simulink model "HILModel"  (Simulink 6.6)
settings: Solver=ode4  StartTime=0.0  StopTime=20  FixedStep=SampleT  RelTol=1e-3
InitFcn:
  | clc
  | Taxi_Var_new
  | failures
  | insInit
  | piccolo_init
values from neighbouring files (symbols this model uses):
  A1 = 0    [Taxi_Var.m]
  Apolar = 0.0899    [Taxi_Var.m]
  CD0 = 0.0219    [Taxi_Var.m]
  chord = S/span    (= 0.384036716878)    [Taxi_Var.m]
  CL0 = 0.1857    [Taxi_Var.m]
  CLa = 4.6206    [Taxi_Var.m]
  CLa_dot = 1.93    [Taxi_Var.m]
  Clb = -0.0043    [Taxi_Var.m]
  ClDa = 0.1695    [Taxi_Var.m]
  CLDe = 0.4032    [Taxi_Var.m]
  CLDf = 0.047    [Taxi_Var.m]
  ClDr = 0.0003    [Taxi_Var.m]
  Clp = -0.4425    [Taxi_Var.m]
  CLq = 8.7465    [Taxi_Var.m]
  Clr = 0.0675    [Taxi_Var.m]
  Cm0 = -0.0902    [Taxi_Var.m]
  Cma = -1.3995    [Taxi_Var.m]
  CmDe = -0.9493    [Taxi_Var.m]
  CmDf = -.021    (= -0.021)    [Taxi_Var.m]
  Cmq = -10.8760    (= -10.876)    [Taxi_Var.m]
  Cnb = 0.0281    [Taxi_Var.m]
  CnDa = -0.0031    [Taxi_Var.m]
  CnDr = -0.0882    [Taxi_Var.m]
  Cnp = -0.0695    [Taxi_Var.m]
  Cnr = -0.1045    [Taxi_Var.m]
  CYb = -0.1999    [Taxi_Var.m]
  CYDr = 0.0192    [Taxi_Var.m]
  damax = 25*deg2rad    (= 0.436332312999)    [Taxi_Var.m]
  damin = -25*deg2rad    (= -0.436332312999)    [Taxi_Var.m]
  datrim = 0*deg2rad    (= 0)    [Taxi_Var.m]
  demax = 15*deg2rad    (= 0.261799387799)    [Taxi_Var.m]
  demin = -15*deg2rad    (= -0.261799387799)    [Taxi_Var.m]
  detrim = -2.4137*deg2rad    (= -0.0421270121554)    [Taxi_Var.m]
  dfland = 30*deg2rad    (= 0.523598775598)    [Taxi_Var.m]
  dfmax = 30*deg2rad    (= 0.523598775598)    [Taxi_Var.m]
  dfmin = 0*deg2rad    (= 0)    [Taxi_Var.m]
  drmax = 25*deg2rad    (= 0.436332312999)    [Taxi_Var.m]
  drmin = -25*deg2rad    (= -0.436332312999)    [Taxi_Var.m]
  drtrim = 0*deg2rad    (= 0)    [Taxi_Var.m]
  dtmax = 1    [Taxi_Var.m]
  dtmin = 0    [Taxi_Var.m]
  dttrim = 0.0725    [Taxi_Var.m]
  Euler_0 = [0; 0; 45]'*pi/180    [Taxi_Var.m]    (also in hilInit.m = [0; 0; 0*pi/180]')
  ISA_g = 9.815    [Taxi_Var.m]
  ISA_hmax = 2000    [Taxi_Var.m]
  ISA_lapse = .0065    (= 0.0065)    [Taxi_Var.m]
  ISA_P0 = 101325    [Taxi_Var.m]
  ISA_R = 287    [Taxi_Var.m]
  ISA_rho0 = 1.225    [Taxi_Var.m]
  ISA_T0 = 289    [Taxi_Var.m]
  Ixx = 3.689084    [Taxi_Var.m]
  Iyy = 7.43789    [Taxi_Var.m]
  Izz = 10.22202    [Taxi_Var.m]
  mass = 22.5    [Taxi_Var.m]
  MinThK = 0.075    [Taxi_Var.m]
  Pos_0 = [0; 0; 1000]'    [Taxi_Var.m]    (also in hilInit.m = [500; 750; 350]')
  PQR_0 = [0; 0; 0]'    [Taxi_Var.m]
  span = 2.3368    [Taxi_Var.m]
  TFact = 0.4    [Taxi_Var.m]
  ThK = 2.18    [Taxi_Var.m]
  Vb_0 = [35; 0; 0]'    [Taxi_Var.m]
undefined symbols (not defined in the file or in its folder): clock, Earth, IdxCmdOrbitRadius, IdxCmdOrbitSense, IdxCmdWp1Alt, IdxCmdWp1Lat, IdxCmdWp1Lon, IdxCmdWp2Alt, IdxCmdWp2Lat, IdxCmdWp2Lon, IdxEstimReserved1, IdxEstimWEast, IdxEstimWNorth, IdxGainsAltD, IdxGainsAltI, IdxGainsAltP, IdxGainsPdynD, IdxGainsPdynI, IdxGainsPdynP, IdxGainsPitchD, IdxGainsPitchI, IdxGainsPitchP, IdxGainsRollD, IdxGainsRollI, IdxGainsRollP, IdxGainsSlopeElevatorD, IdxGainsSlopeElevatorP, IdxGainsTrackConv, IdxGainsTrackD, IdxGainsTrackI, IdxGainsTrackP, IdxGainsTurnD, IdxGainsTurnI, IdxGainsTurnP, IdxGainsYawD, IdxGainsYawI, IdxGainsYawP, IdxLimitsAileronMax, IdxLimitsAileronMin, IdxLimitsBankMax, IdxLimitsBankMin, IdxLimitsElevatorMax, IdxLimitsElevatorMin, IdxLimitsFlapMax, IdxLimitsFlapMin, IdxLimitsPdynMax, IdxLimitsPdynMin, IdxLimitsRudderMax, IdxLimitsRudderMin, IdxLimitsThrottleMax, IdxLimitsThrottleMin, IdxSensorsAlt, IdxSensorsLat, IdxSensorsLon, IdxSensorsVDown, IdxSensorsVEast, IdxSensorsVNorth, IdxStatesGlobal, IdxStatesManual, IdxStatesMode ... (+3)
libraries: piccolo_library x60, simulink x32, aerolibasang x5, aerolibconvert2 x5, aerosimlib x3, aerolibtransform2 x2, aerolibnav x2, xpclib x1, aerolibatmos2 x1, dspmtrx3 x1
(part 3 of 4)

== system HILModel/Autopilot/Autopilot/Altitude Control Vector Inputs/Integral Gain  Scheduling ==
  note: 3. Then the IntegralGain2 = IntegralGain * GainScheduleFactor
  note: 2. We compute GainScheduleFactor = exp(-error^2 / (2*sigma^2))
  note: 1. We compute sigma = ScalingParam * ActuatorRange/2 / Kp
  note: Integral gain scheduling based on a Gaussian distribution, as a function of the error, actuator range, and proportional gain.
  err : Inport
  Gains : Inport  Port=2
  Limits : Inport  Port=3
  Demux : Demux  Outputs=2
  Demux1 : Demux  Outputs=3
  Gain : Gain  Gain=0.5  SaturateOnIntegerOverflow=on
  Gain1 : Gain  Gain=2  SaturateOnIntegerOverflow=on
  Gain2 : Gain  Gain=-1  SaturateOnIntegerOverflow=on
  Math Function : Math  Operator=square  OutDataType=fixdt(1,16,0)  OutScaling=[]  SaturateOnIntegerOverflow=on
  Math Function1 : Math  Operator=square  OutDataType=fixdt(1,16,0)  OutScaling=[]  SaturateOnIntegerOverflow=on
  Math Function2 : Math  OutDataType=fixdt(1,16,0)  OutScaling=[]  SaturateOnIntegerOverflow=on
  Mux1 : Mux  Inputs=3
  Product : Product  Inputs=/**  SaturateOnIntegerOverflow=on
  Product1 : Product  Inputs=*/  SaturateOnIntegerOverflow=on
  Product2 : Product  SaturateOnIntegerOverflow=on
  Scaling param : Constant  Value=0.5
  Sum : Sum  Inputs=+-  SaturateOnIntegerOverflow=on
  Zero Protect : piccolo_library/Math/Zero Protect  SystemSampleTime=-1  p=1  tol=1e-6
  Gains2 : Outport  OutDataType=fixdt(1,16,0)  OutScaling=[]
  wires:
  Zero Protect/1 -> Product/1
  Demux1/1 -> Mux1/1, Zero Protect/1
  Demux1/3 -> Mux1/3
  Product2/1 -> Mux1/2
  Mux1/1 -> Gains2/1
  Demux1/2 -> Product2/2
  Gains/1 -> Demux1/1
  Math Function2/1 -> Product2/1
  Product1/1 -> Math Function2/1
  Gain1/1 -> Product1/2
  Gain2/1 -> Product1/1
  Math Function1/1 -> Gain2/1
  err/1 -> Math Function1/1
  Math Function/1 -> Gain1/1
  Product/1 -> Math Function/1
  Scaling param/1 -> Product/3
  Gain/1 -> Product/2
  Sum/1 -> Gain/1
  Demux/2 -> Sum/2
  Demux/1 -> Sum/1
  Limits/1 -> Demux/1

== system HILModel/Autopilot/Autopilot/Altitude Control Vector Inputs/Min alt ==
  note: Determin the min altitude to use. Either -10000 or the passed in value, depending on if Auto land is enabled
  Globals : Inport
  MinAlt : Inport  Port=2
  -10000 : Constant  Value=-10000
  Climbout : Constant  Value=0
  Convert to 1 based : Constant  Value=1.1
  Default : Constant  Value=0
  Demux : Demux  Outputs=3
  Final Approach : Constant
  Flying : Constant  Value=0
  Land pattern : Constant
  Loop on or off : Switch  Threshold=0.5  SaturateOnIntegerOverflow=on
  Min alt on/off : MultiPortSwitch  Inputs=8  SaturateOnIntegerOverflow=on  InputSameDT=on
  Pre launch : Constant  Value=0
  Sum : Sum  Inputs=++|  SaturateOnIntegerOverflow=on  InputSameDT=on
  Terminator : Terminator
  Terminator1 : Terminator
  Touchdown : Constant
  Transition : Constant  Value=0
  MinAltOut : Outport  OutDataType=fixdt(1,16,0)  OutScaling=[]
  wires:
  Sum/1 -> Min alt on/off/1
  Default/1 -> Min alt on/off/9
  Touchdown/1 -> Min alt on/off/8
  Final Approach/1 -> Min alt on/off/7
  Land pattern/1 -> Min alt on/off/6
  Flying/1 -> Min alt on/off/5
  Transition/1 -> Min alt on/off/3
  Climbout/1 -> Min alt on/off/4
  Pre launch/1 -> Min alt on/off/2
  -10000/1 -> Loop on or off/1
  Min alt on/off/1 -> Loop on or off/2
  Loop on or off/1 -> MinAltOut/1
  Globals/1 -> Demux/1
  Demux/1 -> Terminator1/1
  MinAlt/1 -> Loop on or off/3
  Demux/2 -> Sum/2
  Convert to 1 based/1 -> Sum/1
  Demux/3 -> Terminator/1

== system HILModel/Autopilot/Autopilot/Altitude Control Vector Inputs/PID Controller ==
  note: Standard PID feedback controller with integrator saturation. There are three gains, and three states, one for each term
  Input : Inport
  Cmd : Inport  Port=2
  State : Inport  Port=3
  Gains : Inport  Port=4
  Limits : Inport  Port=5
  IniCond : Inport  Port=6
  Demux : Demux  Outputs=3
  Demux1 : Demux  Outputs=3
  Derivative Gain : Product  Inputs=3  SaturateOnIntegerOverflow=on  InputSameDT=on
  Extended Integrator : Subsystem  AncestorBlock=piccolo_library/Integrators/Extended Integrator  mask(Extended Integrator){T=tsamp}
      mask prompts: T "Sample time:"
      mask help:
      | Trapezoidal integration with integrator reset and anti-windup logic
      | The block computes the integral.  The integrator gets the IC value
      | whenever the enable line is down.  Anytime the enable line is
      | down the output is the IC value.  If the gain goes to zero then the
      | integrator value is reset.
  Proportional Gain : Product  Inputs=3  SaturateOnIntegerOverflow=on  InputSameDT=on
  Scope1 : Scope  NumInputPorts=3
      settings: YMin=0.045~0.038~-1  YMax=0.051~0.058~1  SaveName=ScopeData32
  Scope2 : Scope  NumInputPorts=3
      settings: YMin=0.045~0.038~-1  YMax=0.051~0.058~1  SaveName=ScopeData20
  Sum : Sum  Inputs=|+-  SaturateOnIntegerOverflow=on
  Sum3 : Sum  Inputs=+++  SaturateOnIntegerOverflow=on  InputSameDT=on
  dx/dt with TD : piccolo_library/Derivatives/dx//dt with TD  SystemSampleTime=-1  tsamp=tsamp  tdelay=tdelay
  Output : Outport  OutDataType=fixdt(1,16,0)  OutScaling=[]
  wires:
  Sum3/1 -> Output/1
  Demux1/3 -> Derivative Gain/3
  Demux1/2 -> Extended Integrator/3(Enable)
  Demux1/1 -> Proportional Gain/3
  State/1 -> Demux1/1
  IniCond/1 -> Extended Integrator/2(IniCond)
  Limits/1 -> Extended Integrator/5(Limits)
  Demux/2 -> Extended Integrator/4(Gain)
  Extended Integrator/1(Out) -> Sum3/2, Scope2/2
  Derivative Gain/1 -> Sum3/3, Scope2/3
  Proportional Gain/1 -> Sum3/1, Scope2/1
  Demux/3 -> Derivative Gain/2
  Demux/1 -> Proportional Gain/2
  Gains/1 -> Demux/1
  dx/dt with TD/1 -> Derivative Gain/1
  Sum/1 -> Extended Integrator/1(Input), dx/dt with TD/1, Proportional Gain/1
  Cmd/1 -> Sum/2, Scope1/1, Scope1/2
  Input/1 -> Sum/1

== system HILModel/Autopilot/Autopilot/Altitude Control Vector Inputs/Total Energy1 ==
  TAS : Inport
  Alt : Inport  Port=2
  TASCmd : Inport  Port=3
  AltCmd : Inport  Port=4
  State : Inport  Port=5
  1/2 : Constant  Value=0.5
  Kinetic : Product  Inputs=***  SaturateOnIntegerOverflow=on  InputSameDT=on
  Kinetic1 : Product  Inputs=*/  SaturateOnIntegerOverflow=on  InputSameDT=on
  Kinetic2 : Product  Inputs=***  SaturateOnIntegerOverflow=on  InputSameDT=on
  Sum1 : Sum  SaturateOnIntegerOverflow=on  InputSameDT=on
  Sum2 : Sum  SaturateOnIntegerOverflow=on  InputSameDT=on
  Switch : Switch  Threshold=0.5  SaturateOnIntegerOverflow=on
  Switch1 : Switch  Threshold=0.5  SaturateOnIntegerOverflow=on
  Zero : Constant  Value=0.0
  g1 : Constant  Value=9.806
  Energy : Outport  OutDataType=fixdt(1,16,0)  OutScaling=[]
  Cmd : Outport  Port=2  OutDataType=fixdt(1,16,0)  OutScaling=[]
  wires:
  TASCmd/1 -> Kinetic2/3, Kinetic2/2
  Sum1/1 -> Cmd/1
  AltCmd/1 -> Sum1/2
  Switch1/1 -> Sum1/1
  Kinetic2/1 -> Switch1/1
  Sum2/1 -> Energy/1
  Alt/1 -> Sum2/1
  Switch/1 -> Sum2/2
  Kinetic1/1 -> Kinetic2/1, Kinetic/3
  1/2/1 -> Kinetic1/1
  g1/1 -> Kinetic1/2
  Kinetic/1 -> Switch/1
  State/1 -> Switch/2, Switch1/2
  Zero/1 -> Switch/3, Switch1/3
  TAS/1 -> Kinetic/1, Kinetic/2

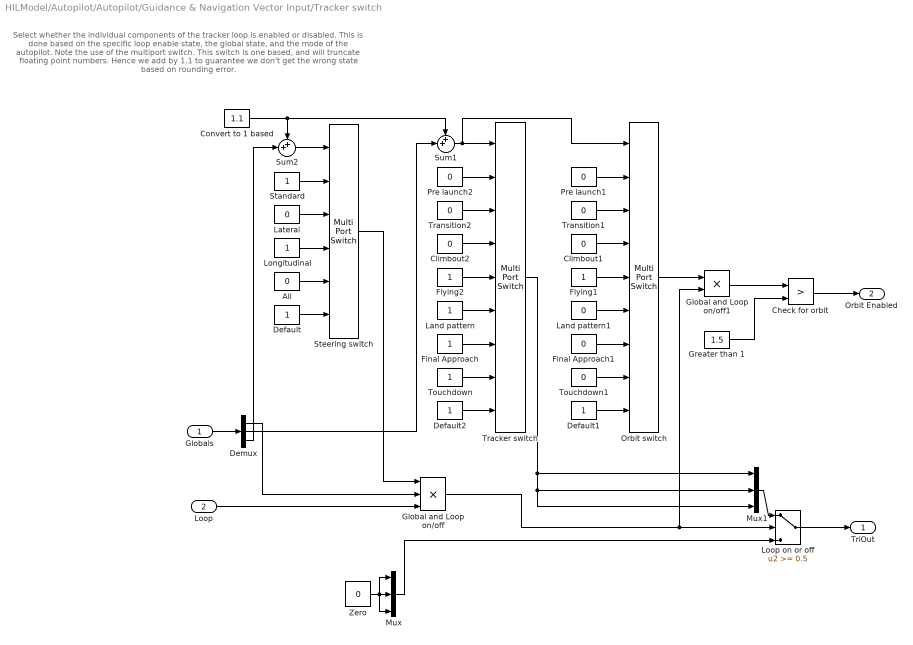
== system HILModel/Autopilot/Autopilot/Guidance & Navigation Vector Input/Tracker switch ==
  note: Select whether the individual components of the tracker loop is enabled or
      | disabled.  This is done based on the specific loop enable state, the global state, and the mode of the autopilot.
      |
      | Note the use of the multiport  switch.  This switch is one based, and will truncate floating point
      | numbers.  Hence we add by 1.1 to guarantee we don't get the wrong state based on rounding
      | error.
  Globals : Inport
  Loop : Inport  Port=2
  All : Constant  Value=0
  Check for orbit : RelationalOperator  Operator=>
  Climbout1 : Constant  Value=0
  Climbout2 : Constant  Value=0
  Convert to 1 based : Constant  Value=1.1
  Default : Constant
  Default1 : Constant
  Default2 : Constant
  Demux : Demux  Outputs=3
  Final Approach : Constant
  Final Approach1 : Constant  Value=0
  Flying1 : Constant
  Flying2 : Constant
  Global and Loop on/off : Product  Inputs=3  SaturateOnIntegerOverflow=on
  Global and Loop on/off1 : Product  SaturateOnIntegerOverflow=on
  Greater than 1 : Constant  Value=1.5
  Land pattern : Constant
  Land pattern1 : Constant  Value=0
  Lateral : Constant  Value=0
  Longitudinal : Constant
  Loop on or off : Switch  Threshold=0.5  SaturateOnIntegerOverflow=on
  Mux : Mux  Inputs=3
  Mux1 : Mux  Inputs=3
  Orbit switch : MultiPortSwitch  Inputs=8  SaturateOnIntegerOverflow=on  InputSameDT=on
  Pre launch1 : Constant  Value=0
  Pre launch2 : Constant  Value=0
  Standard : Constant
  Steering switch : MultiPortSwitch  Inputs=5  SaturateOnIntegerOverflow=on  InputSameDT=on
  Sum1 : Sum  Inputs=++|  SaturateOnIntegerOverflow=on  InputSameDT=on
  Sum2 : Sum  Inputs=++|  SaturateOnIntegerOverflow=on  InputSameDT=on
  Touchdown : Constant
  Touchdown1 : Constant  Value=0
  Tracker switch : MultiPortSwitch  Inputs=8  SaturateOnIntegerOverflow=on  InputSameDT=on
  Transition1 : Constant  Value=0
  Transition2 : Constant  Value=0
  Zero : Constant  Value=0
  TriOut : Outport  OutDataType=fixdt(1,16,0)  OutScaling=[]
  Orbit Enabled : Outport  Port=2  OutDataType=fixdt(1,16,0)  OutScaling=[]
  wires:
  Steering switch/1 -> Global and Loop on/off/1
  Demux/1 -> Global and Loop on/off/2
  Loop/1 -> Global and Loop on/off/3
  Sum2/1 -> Steering switch/1
  Default/1 -> Steering switch/6
  All/1 -> Steering switch/5
  Lateral/1 -> Steering switch/3
  Longitudinal/1 -> Steering switch/4
  Standard/1 -> Steering switch/2
  Convert to 1 based/1 -> Sum2/1, Sum1/1
  Default1/1 -> Orbit switch/9
  Touchdown1/1 -> Orbit switch/8
  Final Approach1/1 -> Orbit switch/7
  Land pattern1/1 -> Orbit switch/6
  Flying1/1 -> Orbit switch/5
  Transition1/1 -> Orbit switch/3
  Climbout1/1 -> Orbit switch/4
  Pre launch1/1 -> Orbit switch/2
  Sum1/1 -> Orbit switch/1, Tracker switch/1
  Default2/1 -> Tracker switch/9
  Touchdown/1 -> Tracker switch/8
  Final Approach/1 -> Tracker switch/7
  Land pattern/1 -> Tracker switch/6
  Flying2/1 -> Tracker switch/5
  Transition2/1 -> Tracker switch/3
  Climbout2/1 -> Tracker switch/4
  Pre launch2/1 -> Tracker switch/2
  Mux1/1 -> Loop on or off/1
  Tracker switch/1 -> Mux1/2, Mux1/3, Mux1/1
  Zero/1 -> Mux/3, Mux/2, Mux/1
  Mux/1 -> Loop on or off/3
  Check for orbit/1 -> Orbit Enabled/1
  Greater than 1/1 -> Check for orbit/2
  Orbit switch/1 -> Global and Loop on/off1/1
  Global and Loop on/off1/1 -> Check for orbit/1
  Demux/3 -> Sum2/2
  Demux/2 -> Sum1/2
  Global and Loop on/off/1 -> Global and Loop on/off1/2, Loop on or off/2
  Globals/1 -> Demux/1
  Loop on or off/1 -> TriOut/1

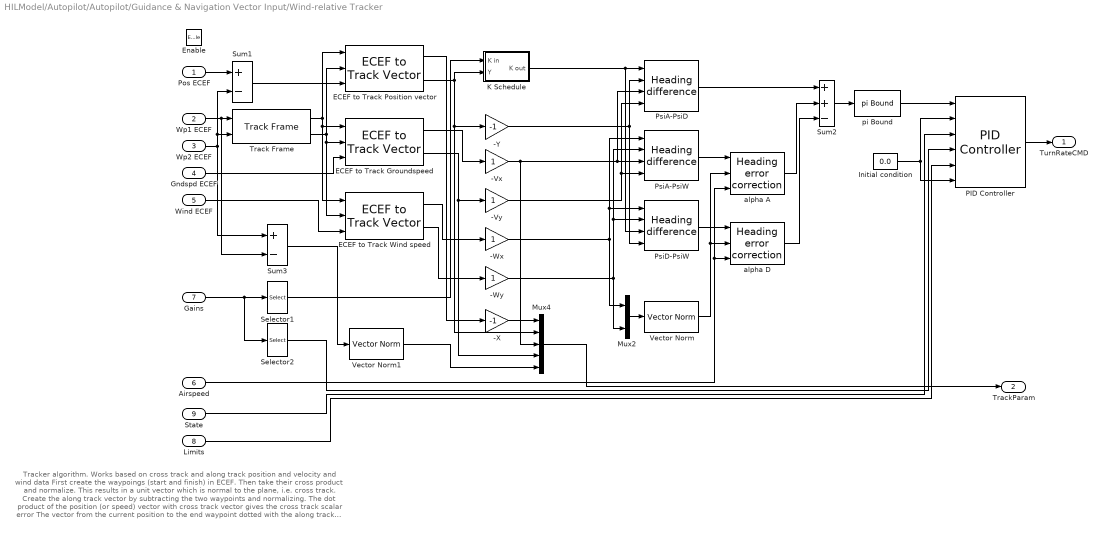
== system HILModel/Autopilot/Autopilot/Guidance & Navigation Vector Input/Wind-relative Tracker ==
  note: Tracker algorithm.  Works based on cross track and along track position and velocity and wind data
      |
      | First create the waypoings (start and finish) in ECEF.  Then take their cross product and normalize.  This results in a unit vector which is normal to the plane, i.e. cross track.
      | Create the along track vector by subtracting the two waypoints and normalizing.
      | The dot product of the position (or speed) vector with cross track vector gives the cross track scalar error
      | The vector from the current position to the end waypoint dotted with the along track vector gives the along track value
  Pos ECEF : Inport
  Wp1 ECEF : Inport  Port=2
  Wp2 ECEF : Inport  Port=3
  Gndspd ECEF : Inport  Port=4
  Wind ECEF : Inport  Port=5
  Airspeed : Inport  Port=6
  Gains : Inport  Port=7
  Limits : Inport  Port=8
  State : Inport  Port=9
  Enable : EnablePort
  -Vx : Gain  SaturateOnIntegerOverflow=on
  -Vy : Gain  SaturateOnIntegerOverflow=on
  -Wx : Gain  SaturateOnIntegerOverflow=on
  -Wy : Gain  SaturateOnIntegerOverflow=on
  -X : Gain  Gain=-1  SaturateOnIntegerOverflow=on
  -Y : Gain  Gain=-1  SaturateOnIntegerOverflow=on
  ECEF to Track Groundspeed : piccolo_library/Transformations/ECEF to Track Vector  SystemSampleTime=-1
  ECEF to Track Position vector : piccolo_library/Transformations/ECEF to Track Vector  SystemSampleTime=-1
  ECEF to Track Wind speed : piccolo_library/Transformations/ECEF to Track Vector  SystemSampleTime=-1
  Initial condition : Constant  Value=0.0
  K Schedule : Subsystem
  Mux2 : Mux  Inputs=2
  Mux4 : Mux  Inputs=5
  PID Controller : piccolo_library/Controllers/PID Controller  SystemSampleTime=-1  tsamp=tsamp  tdelay=tsamp
  PsiA-PsiD : piccolo_library/Controllers/Guidance/Heading difference  SystemSampleTime=-1
  PsiA-PsiW : piccolo_library/Controllers/Guidance/Heading difference  SystemSampleTime=-1
  PsiD-PsiW : piccolo_library/Controllers/Guidance/Heading difference  SystemSampleTime=-1
  Selector1 : Selector  IndexOptions=Index vector (dialog)  Indices=[4]  OutputSizes=1  InputPortWidth=4
  Selector2 : Selector  IndexOptions=Index vector (dialog)  Indices=[1 2 3]  OutputSizes=1  InputPortWidth=4
  Sum1 : Sum  Inputs=+-  SaturateOnIntegerOverflow=on  InputSameDT=on
  Sum2 : Sum  Inputs=++-  SaturateOnIntegerOverflow=on  InputSameDT=on
  Sum3 : Sum  Inputs=+-  SaturateOnIntegerOverflow=on  InputSameDT=on
  Track Frame : piccolo_library/Transformations/Track Frame  SystemSampleTime=-1
  Vector Norm : piccolo_library/Math/Vector Norm  SystemSampleTime=-1
  Vector Norm1 : piccolo_library/Math/Vector Norm  SystemSampleTime=-1
  alpha A : piccolo_library/Controllers/Guidance/Heading error correction  SystemSampleTime=-1
  alpha D : piccolo_library/Controllers/Guidance/Heading error correction  SystemSampleTime=-1
  pi Bound : piccolo_library/Math/pi Bound  SystemSampleTime=-1
  TurnRateCMD : Outport  OutDataType=fixdt(1,16,0)  OutScaling=[]
  TrackParam : Outport  Port=2  OutDataType=fixdt(1,16,0)  OutScaling=[]
  wires:
  Sum3/1 -> Vector Norm1/1
  Vector Norm1/1 -> Mux4/5
  -Y/1 -> PsiD-PsiW/4, PsiA-PsiD/2
  K Schedule/1(K out) -> PsiA-PsiD/1, PsiD-PsiW/3
  PID Controller/1 -> TurnRateCMD/1
  Initial condition/1 -> PID Controller/2, PID Controller/6
  -X/1 -> Mux4/1
  ECEF to Track Wind speed/1 -> -Wx/1
  ECEF to Track Wind speed/2 -> -Wy/1
  ECEF to Track Groundspeed/2 -> Mux4/4, -Vy/1
  ECEF to Track Groundspeed/1 -> -Vx/1
  ECEF to Track Position vector/1 -> -X/1
  ECEF to Track Position vector/2 -> -Y/1, Mux4/2, K Schedule/2(Y)
  Selector1/1 -> K Schedule/1(K in)
  Mux2/1 -> Vector Norm/1
  Vector Norm/1 -> alpha D/2, alpha A/2
  -Wy/1 -> Mux2/2, PsiD-PsiW/2, PsiA-PsiW/2
  -Vy/1 -> PsiA-PsiD/4, PsiA-PsiW/4
  -Wx/1 -> Mux2/1, PsiD-PsiW/1, PsiA-PsiW/1
  -Vx/1 -> Mux4/3, PsiA-PsiD/3, PsiA-PsiW/3
  pi Bound/1 -> PID Controller/1
  Sum2/1 -> pi Bound/1
  alpha D/1 -> Sum2/3
  alpha A/1 -> Sum2/2
  PsiA-PsiD/1 -> Sum2/1
  Limits/1 -> PID Controller/5
  State/1 -> PID Controller/3
  PsiD-PsiW/1 -> alpha D/1
  PsiA-PsiW/1 -> alpha A/1
  Mux4/1 -> TrackParam/1
  Selector2/1 -> PID Controller/4
  Airspeed/1 -> alpha D/3, alpha A/3
  Gains/1 -> Selector2/1, Selector1/1
  Wind ECEF/1 -> ECEF to Track Wind speed/3
  Gndspd ECEF/1 -> ECEF to Track Groundspeed/3
  Track Frame/2 -> ECEF to Track Wind speed/2, ECEF to Track Groundspeed/2, ECEF to Track Position vector/2
  Track Frame/1 -> ECEF to Track Wind speed/1, ECEF to Track Groundspeed/1, ECEF to Track Position vector/1
  Sum1/1 -> ECEF to Track Position vector/3
  Pos ECEF/1 -> Sum1/1
  Wp2 ECEF/1 -> Sum3/1, Sum1/2, Track Frame/2
  Wp1 ECEF/1 -> Sum3/2, Track Frame/1

== system HILModel/Autopilot/Autopilot/Pitch Control  Vector Inputs/PDynCmd ==
  AltError : Inport
  QCmd : Inport  Port=2
  QShift : Inport  Port=3
  QLimits : Inport  Port=4
  States : Inport  Port=5
  Density : Inport  Port=6
  -0.2 : Gain  Gain=-.2  SaturateOnIntegerOverflow=on
  0.3 : Gain  Gain=.3  SaturateOnIntegerOverflow=on
  1-based : Constant  Value=1.1
  All : Constant  Value=0
  Default : Constant  Value=0
  Enabled? : Logic  AllPortsSameDT=off
  Energy or not? : Switch  Threshold=0.5  SaturateOnIntegerOverflow=on
  Gravity : Gain  Gain=9.8  SaturateOnIntegerOverflow=on
  Lateral : Constant
  Limited QShift : piccolo_library/Nonlinear/SaturationEx  SystemSampleTime=-1
  Longitudinal : Constant  Value=0
  Manual assist switch : MultiPortSwitch  Inputs=5  SaturateOnIntegerOverflow=on  InputSameDT=on
  Mux : Mux  Inputs=2
  PDyn saturation : piccolo_library/Nonlinear/SaturationEx  SystemSampleTime=-1
  PDyn saturation1 : piccolo_library/Nonlinear/SaturationEx  SystemSampleTime=-1
  Qshift : Product  SaturateOnIntegerOverflow=on
  Selector1 : Selector  IndexOptions=Index vector (dialog)  Indices=IdxStatesManual  OutputSizes=1  InputPortWidth=SizeStates
  Selector2 : Selector  IndexOptions=Index vector (dialog)  Indices=IdxStatesAltToPdyn  OutputSizes=1  InputPortWidth=SizeStates
  Standard : Constant
  Sum : Sum  Inputs=|++  SaturateOnIntegerOverflow=on
  Sum1 : Sum  SaturateOnIntegerOverflow=on
  QCmdOut : Outport  OutDataType=fixdt(1,16,0)  OutScaling=[]
  QCmdNom : Outport  Port=2  OutDataType=fixdt(1,16,0)  OutScaling=[]
  wires:
  Enabled?/1 -> Energy or not?/2
  Manual assist switch/1 -> Enabled?/1
  Selector2/1 -> Enabled?/2
  PDyn saturation1/1 -> QCmdNom/1
  Sum1/1 -> PDyn saturation/1
  Energy or not?/1 -> Sum1/2
  QLimits/1 -> PDyn saturation1/2, PDyn saturation/2
  PDyn saturation/1 -> QCmdOut/1
  QShift/1 -> Energy or not?/3
  Limited QShift/1 -> Energy or not?/1
  Sum/1 -> Manual assist switch/1
  1-based/1 -> Sum/2
  Selector1/1 -> Sum/1
  States/1 -> Selector2/1, Selector1/1
  Default/1 -> Manual assist switch/6
  All/1 -> Manual assist switch/5
  Lateral/1 -> Manual assist switch/3
  Longitudinal/1 -> Manual assist switch/4
  Standard/1 -> Manual assist switch/2
  QCmd/1 -> PDyn saturation1/1, Sum1/1, -0.2/1, 0.3/1
  Qshift/1 -> Limited QShift/1
  Mux/1 -> Limited QShift/2
  0.3/1 -> Mux/2
  -0.2/1 -> Mux/1
  Gravity/1 -> Qshift/1
  AltError/1 -> Gravity/1
  Density/1 -> Qshift/2

== system HILModel/Autopilot/Autopilot/Pitch Control  Vector Inputs/Pdyn Hold ==
  Input : Inport
  Cmd : Inport  Port=2
  State : Inport  Port=3
  Gains : Inport  Port=4
  Limits : Inport  Port=5
  Actuator Trim : Inport  Port=6
  50 [Pa/s] : Constant  Value=100
  PID Controller : Subsystem  AncestorBlock=piccolo_library/Controllers/PID Controller  mask(PID Controller){tsamp=tsamp, tdelay=0.5}
      mask prompts: tsamp "Sample time:"; tdelay "Time derivative delay:"
      mask help: Generic PID (proportional, integral, derivative) controller with a single input and a single output.
  Rate Limit Ex : piccolo_library/Nonlinear/Rate Limit Ex  SystemSampleTime=-1  T=tsamp
  Out : Outport  OutDataType=fixdt(1,16,0)  OutScaling=[]
  wires:
  Actuator Trim/1 -> PID Controller/6(IniCond)
  Limits/1 -> PID Controller/5(Limits)
  Gains/1 -> PID Controller/4(Gains)
  State/1 -> PID Controller/3(State)
  PID Controller/1(Output) -> Out/1
  Rate Limit Ex/1 -> PID Controller/2(Cmd)
  Input/1 -> PID Controller/1(Input)
  50 [Pa/s]/1 -> Rate Limit Ex/2
  Cmd/1 -> Rate Limit Ex/1

== system HILModel/Autopilot/Autopilot/Pitch Control  Vector Inputs/Pitch Angle Hold ==
  note: Controller which takes in pitch rate and pitch angle and outputs elevator. The integral term is not used. Yet.
  Pitch angle : Inport
  Pitch rate : Inport  Port=2
  Pitch angle cmd : Inport  Port=3
  Pitch rate cmd : Inport  Port=4
  State : Inport  Port=5
  Gains : Inport  Port=6
  Demux1 : Demux  Outputs=3
  Demux5 : Demux  Outputs=3
  Derivative Gain : Product  Inputs=3  SaturateOnIntegerOverflow=on  InputSameDT=on
  Low-pass Filter : piccolo_library/Filters/Low-pass Filter  SystemSampleTime=-1  f=3  t=tsamp
  Proportional Gain : Product  Inputs=3  SaturateOnIntegerOverflow=on  InputSameDT=on
  Scope : Scope  NumInputPorts=5
      settings: YMin=-1~-0.075~-0.075~-5e+006~-5e+006  YMax=1~0.1~0.1~3.5e+007~3.5e+007  SaveName=ScopeData5
  Sum : Sum  SaturateOnIntegerOverflow=on  InputSameDT=on
  Sum1 : Sum  Inputs=|+-  SaturateOnIntegerOverflow=on  InputSameDT=on
  Sum2 : Sum  Inputs=|+-  SaturateOnIntegerOverflow=on  InputSameDT=on
  Terminator : Terminator
  Terminator1 : Terminator
  Out : Outport  OutDataType=fixdt(1,16,0)  OutScaling=[]
  wires:
  Demux1/2 -> Terminator1/1
  Demux1/1 -> Proportional Gain/3
  Demux1/3 -> Derivative Gain/3
  State/1 -> Demux1/1
  Demux5/2 -> Terminator/1
  Sum/1 -> Out/1, Scope/4
  Derivative Gain/1 -> Sum/2
  Proportional Gain/1 -> Sum/1, Scope/5
  Demux5/3 -> Derivative Gain/2
  Low-pass Filter/1 -> Derivative Gain/1
  Demux5/1 -> Proportional Gain/2
  Sum2/1 -> Proportional Gain/1, Scope/3
  Sum1/1 -> Low-pass Filter/1
  Pitch angle cmd/1 -> Sum2/2, Scope/1
  Pitch angle/1 -> Sum2/1, Scope/2
  Gains/1 -> Demux5/1
  Pitch rate/1 -> Sum1/1
  Pitch rate cmd/1 -> Sum1/2

== system HILModel/Autopilot/Autopilot/Roll Control Vector Inputs/Bank Angle Hold ==
  note: Controller which takes in roll rate and roll angle and outputs aileron.  Note that the derivative
      | term is simply the roll rate rather than the derivative of the error signal.
      | This is for backward compatible systems which aren't using the attitude data.
  note: pid
  Roll Rate : Inport
  Roll Angle : Inport  Port=2
  Cmd : Inport  Port=3
  State : Inport  Port=4
  Gains : Inport  Port=5
  Limits : Inport  Port=6
  IniCond : Inport  Port=7
  Demux1 : Demux  Outputs=3
  Demux2 : Demux  Outputs=3
  Derivative Gain : Product  Inputs=3  SaturateOnIntegerOverflow=on  InputSameDT=on
  Extended Integrator : piccolo_library/Integrators/Extended Integrator  SystemSampleTime=-1  T=tsamp
  Low-pass Filter : piccolo_library/Filters/Low-pass Filter  SystemSampleTime=-1  f=3  t=tsamp
  Proportional Gain : Product  Inputs=3  SaturateOnIntegerOverflow=on  InputSameDT=on
  Scope : Scope  NumInputPorts=10
      settings: YMin=-1~-0.07~-0.07~-0.02~-1~-1~-1~-1~-1~-1  YMax=1~0.03~0.03~0.07~1~1~1~1~1~1
  Sum2 : Sum  Inputs=+++  SaturateOnIntegerOverflow=on  InputSameDT=on
  Sum3 : Sum  Inputs=|+-  SaturateOnIntegerOverflow=on  InputSameDT=on
  Out : Outport  OutDataType=fixdt(1,16,0)  OutScaling=[]
  wires:
  Demux2/3 -> Derivative Gain/3
  Demux2/2 -> Extended Integrator/3
  Demux2/1 -> Proportional Gain/3
  State/1 -> Demux2/1
  Roll Rate/1 -> Low-pass Filter/1
  Low-pass Filter/1 -> Derivative Gain/1
  Demux1/2 -> Extended Integrator/4
  Sum2/1 -> Out/1, Scope/4
  Derivative Gain/1 -> Sum2/3, Scope/6  "derv"
  Extended Integrator/1 -> Sum2/2, Scope/5  "int"
  Proportional Gain/1 -> Sum2/1
  Demux1/3 -> Derivative Gain/2
  Demux1/1 -> Proportional Gain/2
  Limits/1 -> Extended Integrator/5
  IniCond/1 -> Extended Integrator/2
  Sum3/1 -> Extended Integrator/1, Proportional Gain/1, Scope/3  "err"
  Gains/1 -> Demux1/1
  Roll Angle/1 -> Scope/2, Sum3/1  "roll"
  Cmd/1 -> Sum3/2, Scope/1  "cmd"

== system HILModel/Autopilot/Autopilot/Roll Control Vector Inputs/Damper switch ==
  note: Select whether the individual components of the pitch and roll damper  loops are enabled or disabled.
      | This is done based on the specific loop enable state, the global state, and the mode of the autopilot.
      |
      | Note the use of the multiport  switch.  This switch is one based, and will truncate floating point
      | numbers.  Hence we add by 1.1 to guarantee we don't get the wrong state based on rounding
      | error.
  Globals : Inport
  Loop : Inport  Port=2
  Climbout : Constant
  Convert to 1 based : Constant  Value=1.1
  Default : Constant
  Demux : Demux  Outputs=3
  Display1 : Display
  Display2 : Display
  Display3 : Display
  Final Approach : Constant
  Flying : Constant
  Global and Loop on/off : Product  SaturateOnIntegerOverflow=on
  Land pattern : Constant
  Loop on or off : Switch  Threshold=0.5  SaturateOnIntegerOverflow=on
  Mux : Mux  Inputs=3
  Mux1 : Mux  Inputs=3
  Pre launch : Constant  Value=0
  Proportional\ Integral switch : MultiPortSwitch  Inputs=8  SaturateOnIntegerOverflow=on  InputSameDT=on
  Sum : Sum  Inputs=++|  SaturateOnIntegerOverflow=on  InputSameDT=on
  Terminator : Terminator
  Touchdown : Constant
  Transition : Constant  Value=0
  Zero : Constant  Value=0
  TriOut : Outport  OutDataType=fixdt(1,16,0)  OutScaling=[]
  wires:
  Default/1 -> Proportional\ Integral switch/9
  Touchdown/1 -> Proportional\ Integral switch/8
  Demux/3 -> Terminator/1
  Mux1/1 -> Loop on or off/1
  Proportional\ Integral switch/1 -> Mux1/3, Mux1/2, Mux1/1
  Final Approach/1 -> Proportional\ Integral switch/7
  Land pattern/1 -> Proportional\ Integral switch/6
  Flying/1 -> Proportional\ Integral switch/5
  Transition/1 -> Proportional\ Integral switch/3
  Climbout/1 -> Proportional\ Integral switch/4
  Pre launch/1 -> Proportional\ Integral switch/2
  Convert to 1 based/1 -> Sum/1
  Demux/2 -> Sum/2
  Sum/1 -> Proportional\ Integral switch/1
  Global and Loop on/off/1 -> Loop on or off/2, Display2/1
  Loop/1 -> Global and Loop on/off/2, Display3/1
  Demux/1 -> Global and Loop on/off/1, Display1/1
  Globals/1 -> Demux/1
  Zero/1 -> Mux/3, Mux/2, Mux/1
  Mux/1 -> Loop on or off/3
  Loop on or off/1 -> TriOut/1

== system HILModel/Autopilot/Autopilot/Roll Control Vector Inputs/Turn Rate Hold ==
  note: Standard PID feedback controller with integrator saturation. There are three gains, and three states, one for each term
  Input : Inport
  Cmd : Inport  Port=2
  State : Inport  Port=3
  Gains : Inport  Port=4
  Limits : Inport  Port=5
  IniCond : Inport  Port=6
  Demux : Demux  Outputs=3
  Demux1 : Demux  Outputs=3
  Derivative Gain : Product  Inputs=3  SaturateOnIntegerOverflow=on  InputSameDT=on
  Extended Integrator : piccolo_library/Integrators/Extended Integrator  SystemSampleTime=-1  T=tsamp
  Proportional Gain : Product  Inputs=3  SaturateOnIntegerOverflow=on  InputSameDT=on
  Scope1 : Scope  NumInputPorts=5
      settings: YMin=0.09325~0.09~-0.005~-1~-1  YMax=0.09475~0.1075~0.0125~1~1  SaveName=ScopeData25
  Sum : Sum  Inputs=|+-  SaturateOnIntegerOverflow=on
  Sum3 : Sum  Inputs=+++  SaturateOnIntegerOverflow=on  InputSameDT=on
  dx/dt with TD : piccolo_library/Derivatives/dx//dt with TD  SystemSampleTime=-1  tsamp=tsamp  tdelay=tdelay
  Output : Outport  OutDataType=fixdt(1,16,0)  OutScaling=[]
  wires:
  Sum3/1 -> Output/1, Scope1/4
  Demux1/3 -> Derivative Gain/3
  Demux1/2 -> Extended Integrator/3
  Demux1/1 -> Proportional Gain/3
  State/1 -> Demux1/1
  IniCond/1 -> Extended Integrator/2
  Limits/1 -> Extended Integrator/5
  Demux/2 -> Extended Integrator/4
  Extended Integrator/1 -> Sum3/2
  Derivative Gain/1 -> Sum3/3
  Proportional Gain/1 -> Sum3/1
  Demux/3 -> Derivative Gain/2
  Demux/1 -> Proportional Gain/2
  Gains/1 -> Demux/1
  dx/dt with TD/1 -> Derivative Gain/1
  Sum/1 -> Extended Integrator/1, dx/dt with TD/1, Scope1/3, Proportional Gain/1
  Cmd/1 -> Sum/2, Scope1/1
  Input/1 -> Sum/1, Scope1/2

== system HILModel/Autopilot/L1 Adaptive Controller LATERAL-DIRECTIONAL/PF Yaw Channel L1 Augmentation/Adaptive Law ==
  u_psi_tilda : Inport
  Integrator : Integrator  LimitOutput=on  UpperSaturationLimit=Pbound  LowerSaturationLimit=-Pbound
  ON : Constant  Value=gamma
  Projection : Product  RndMeth=Zero
  Scope1 : Scope  NumInputPorts=3
      settings: YMin=-0.1~-0.004~-6  YMax=0.1~0.003~8  SaveName=ScopeData27
  sighat_2 : Outport
  wires:
  Integrator/1 -> sighat_2/1, Scope1/1
  ON/1 -> Projection/1
  Projection/1 -> Integrator/1, Scope1/3
  u_psi_tilda/1 -> Projection/2, Scope1/2  "u_psi_tilda"

== system HILModel/Autopilot/L1 Adaptive Controller LATERAL-DIRECTIONAL/PF Yaw Channel L1 Augmentation/C(s) ==
  sighat_2 : Inport
  Integrator2 : Integrator
  ON : Constant  Value=omega
  Product : Product  RndMeth=Zero
  Sum2 : Sum  Inputs=|+-
  C_sighat_2 : Outport
  wires:
  Integrator2/1 -> C_sighat_2/1, Sum2/2
  Sum2/1 -> Product/2
  Product/1 -> Integrator2/1
  sighat_2/1 -> Sum2/1
  ON/1 -> Product/1

== system HILModel/Autopilot/L1 Adaptive Controller LATERAL-DIRECTIONAL/PF Yaw Channel L1 Augmentation/State predictor ==
  u2 : Inport
  sighat_2 : Inport  Port=2
  Integrator2 : Integrator
  ON : Constant  Value=m
  Product : Product  RndMeth=Zero
  Sum1 : Sum  Inputs=|++
  Sum2 : Sum  Inputs=|+-
  u_psi_hat : Outport
  wires:
  sighat_2/1 -> Sum1/2
  Sum1/1 -> Sum2/1
  u2/1 -> Sum1/1
  Integrator2/1 -> u_psi_hat/1, Sum2/2
  Sum2/1 -> Product/2
  Product/1 -> Integrator2/1
  ON/1 -> Product/1

== system HILModel/Autopilot/L1 Adaptive Controller LONGITUDINAL/PF Yaw Channel L1 Augmentation/Adaptive Law ==
  u_psi_tilda : Inport
  Integrator : Integrator  LimitOutput=on  UpperSaturationLimit=Pbound  LowerSaturationLimit=-Pbound
  ON : Constant  Value=gamma
  Projection : Product  RndMeth=Zero
  Scope1 : Scope  NumInputPorts=3
      settings: TimeRange=4  YMin=-0.1~-1000~-6  YMax=0.1~200~8  SaveName=ScopeData27
  sighat_2 : Outport
  wires:
  u_psi_tilda/1 -> Scope1/2, Projection/2  "u_psi_tilda"
  Projection/1 -> Scope1/3, Integrator/1
  ON/1 -> Projection/1
  Integrator/1 -> Scope1/1, sighat_2/1

== system HILModel/Autopilot/L1 Adaptive Controller LONGITUDINAL/PF Yaw Channel L1 Augmentation/C(s) ==
  sighat_2 : Inport
  Integrator2 : Integrator
  ON : Constant  Value=omega
  Product : Product  RndMeth=Zero
  Sum2 : Sum  Inputs=|+-
  C_sighat_2 : Outport
  wires:
  ON/1 -> Product/1
  sighat_2/1 -> Sum2/1
  Product/1 -> Integrator2/1
  Sum2/1 -> Product/2
  Integrator2/1 -> Sum2/2, C_sighat_2/1

== system HILModel/Autopilot/L1 Adaptive Controller LONGITUDINAL/PF Yaw Channel L1 Augmentation/State predictor ==
  u2 : Inport
  sighat_2 : Inport  Port=2
  Integrator2 : Integrator
  ON : Constant  Value=m
  Product : Product  RndMeth=Zero
  Sum1 : Sum  Inputs=|++
  Sum2 : Sum  Inputs=|+-
  u_psi_hat : Outport
  wires:
  ON/1 -> Product/1
  Product/1 -> Integrator2/1
  Sum2/1 -> Product/2
  Integrator2/1 -> Sum2/2, u_psi_hat/1
  u2/1 -> Sum1/1
  Sum1/1 -> Sum2/1
  sighat_2/1 -> Sum1/2

== system HILModel/Plant Model/Generic Sensor/Dynamics/No Dynamics ==
  In1 : Inport
  Out1 : Outport
  wires:
  In1/1 -> Out1/1

== system HILModel/Plant Model/Generic Sensor/Dynamics/Second-order Dynamics ==
  In1 : Inport
  Demux : Demux  Outputs=3
  Mux : Mux  Inputs=3
  Transfer Fcn X : TransferFcn  Numerator=[w_g*w_g]  Denominator="[1 2*z_g*w_g  w_g*w_g]"
  Transfer Fcn Y : TransferFcn  Numerator=[w_g*w_g]  Denominator="[1 2*z_g*w_g  w_g*w_g]"
  Transfer Fcn Z : TransferFcn  Numerator=[w_g*w_g]  Denominator="[1 2*z_g*w_g  w_g*w_g]"
  Out1 : Outport
  wires:
  Transfer Fcn Z/1 -> Mux/3
  Demux/3 -> Transfer Fcn Z/1
  Transfer Fcn Y/1 -> Mux/2
  Demux/2 -> Transfer Fcn Y/1
  Transfer Fcn X/1 -> Mux/1
  Demux/1 -> Transfer Fcn X/1
  Mux/1 -> Out1/1
  In1/1 -> Demux/1

== system HILModel/Plant Model/Plant/6-DOF EOM/Get Euler Dot ==
  p,q,r : Inport
  Euler : Inport  Port=2
  Mux1 : Mux  Inputs=[3 3]
  Mux2 : Mux  Inputs=3
  phidot : Fcn  Expr=u[1]+u[2]*sin(u[4])*tan(u[5])+u[3]*cos(u[4])*tan(u[5])
  psidot : Fcn  Expr=u[2]*sin(u[4])/cos(u[5])+u[3]*cos(u[4])/cos(u[5])
  thetadot : Fcn  Expr=u[2]*cos(u[4])-u[3]*sin(u[4])
  Euler_dot : Outport
  wires:
  Mux2/1 -> Euler_dot/1
  phidot/1 -> Mux2/1
  thetadot/1 -> Mux2/2
  psidot/1 -> Mux2/3
  Mux1/1 -> thetadot/1, phidot/1, psidot/1
  p,q,r/1 -> Mux1/1
  Euler/1 -> Mux1/2

== system HILModel/Plant Model/Plant/6-DOF EOM/RB2LTP ==
  Euler : Inport
  11 : Fcn  Expr=cos(u[3])*cos(u[2])
  12 : Fcn  Expr=sin(u[3])*cos(u[2])
  13 : Fcn  Expr=-sin(u[2])
  21 : Fcn  Expr=cos(u[3])*sin(u[2])*sin(u[1])-sin(u[3])*cos(u[1])
  22 : Fcn  Expr=sin(u[3])*sin(u[2])*sin(u[1])+cos(u[3])*cos(u[1])
  23 : Fcn  Expr=cos(u[2])*sin(u[1])
  31 : Fcn  Expr=cos(u[3])*sin(u[2])*cos(u[1])+sin(u[3])*sin(u[1])
  32 : Fcn  Expr=sin(u[3])*sin(u[2])*cos(u[1])-cos(u[3])*sin(u[1])
  33 : Fcn  Expr=cos(u[2])*cos(u[1])
  Mux2 : Mux  Inputs=9
  Reshape : Reshape  OutputDimensionality=Customize  OutputDimensions=[3,3]
  Rot : Outport
  wires:
  33/1 -> Mux2/9
  32/1 -> Mux2/8
  31/1 -> Mux2/7
  23/1 -> Mux2/6
  22/1 -> Mux2/5
  21/1 -> Mux2/4
  13/1 -> Mux2/3
  12/1 -> Mux2/2
  11/1 -> Mux2/1
  Mux2/1 -> Reshape/1
  Euler/1 -> 11/1, 33/1, 32/1, 31/1, 23/1, 22/1, 21/1, 13/1, 12/1
  Reshape/1 -> Rot/1

== system HILModel/Plant Model/Plant/6-DOF EOM/[V1,2,3,W1,2,3] ==
  note: V*dot =Inv(A){[F ; M] - SigmaAV*}
  "[F ; M]" : Inport
  Euler : Inport  Port=2
  V* : Inport  Port=3  PortDimensions=6
  A = [M ; J] : Subsystem
  Acc_meas : Product  Inputs=/*  Multiplication=Matrix(*)  SaturateOnIntegerOverflow=on  InputSameDT=on
  Demux : Demux  Outputs=[3;3]
  Get Grav Force in Body : Subsystem
  Gravitational Acc : Constant  Value=[0 0 -ISA_g]  VectorParams1D=off
  Reshape1 : Reshape
  Reshape2 : Reshape
  Selector3 : Selector  IndexOptions=Index vector (dialog)  Indices=1:3  OutputSizes=1  InputPortWidth=6
  Sigma : Subsystem
  Sigma*A : Product  Multiplication=Matrix(*)  SaturateOnIntegerOverflow=on  InputSameDT=on
  Sigma*A*V* : Product  Multiplication=Matrix(*)  SaturateOnIntegerOverflow=on  InputSameDT=on
  Sum1 : Sum  Inputs=+-|  SaturateOnIntegerOverflow=on  InputSameDT=on
  Sum2 : Sum  Inputs=++|  SaturateOnIntegerOverflow=on  InputSameDT=on
  Terminator1 : Terminator
  "V*dot " : Product  Inputs=/*  Multiplication=Matrix(*)  SaturateOnIntegerOverflow=on  InputSameDT=on
  "Acc_meas " : Outport
  V*dot : Outport  Port=2
  wires:
  Sum2/1 -> Reshape2/1
  Get Grav Force in Body/1(Grav Force (Body)) -> Reshape1/1
  Selector3/1 -> Sum2/2
  Euler/1 -> Get Grav Force in Body/1(Euler)
  Gravitational Acc/1 -> Get Grav Force in Body/2(Grav Force)
  Acc_meas/1 -> Selector3/1
  Sigma*A/1 -> Sigma*A*V*/1
  "V*dot "/1 -> V*dot/1
  V*/1 -> Demux/1, Sigma*A*V*/2
  Demux/2 -> Sigma/1(pqr)
  Sigma*A*V*/1 -> Sum1/2
  "[F ; M]"/1 -> Acc_meas/2, Sum1/1
  Sigma/1(Sigma) -> Sigma*A/1
  Demux/1 -> Terminator1/1
  A = [M ; J]/1(A Matrix) -> Sigma*A/2, Acc_meas/1, "V*dot "/1
  Sum1/1 -> "V*dot "/2
  Reshape1/1 -> Sum2/1
  Reshape2/1 -> "Acc_meas "/1

== system HILModel/Plant Model/Plant/Engine Model/Get To1 ==
  dt : Inport
  Divide : Product  Inputs=3  OutScaling=2^-10
  Math Function : Math  Operator=pow  SaturateOnIntegerOverflow=on
  Math Function1 : Math  Operator=pow  SaturateOnIntegerOverflow=on
  MaxRPM : Gain  Gain=7200  SaturateOnIntegerOverflow=on
  Min RPM : Constant  Value=2000
  Min Th K : Constant  Value=MinThK
  Prop Diameter (in) : Constant  Value=17
  Prop Diameter (in)1 : Constant  Value=2
  Prop Diameter (in)2 : Constant  Value=4
  Saturation : Saturate  UpperLimit=1.0  LowerLimit=0.2
  Sum : Sum  Inputs=|++
  Sum1 : Sum  Inputs=|++
  TFact : simulink/Math Operations/Slider Gain  SystemSampleTime=-1  low=0  gain=0.2  high=1
  "TFact " : Gain  Gain=TFact  SaturateOnIntegerOverflow=on
  Th K : Gain  Gain=ThK  SaturateOnIntegerOverflow=on
  To Constant : Constant  Value=2.83e-12
  To : Outport
  wires:
  Saturation/1 -> Th K/1
  Prop Diameter (in)1/1 -> Math Function/2
  Prop Diameter (in)2/1 -> Math Function1/2
  Prop Diameter (in)/1 -> Math Function1/1
  Math Function/1 -> Divide/1
  Math Function1/1 -> Divide/2
  To Constant/1 -> Divide/3
  Divide/1 -> TFact/1
  TFact/1 -> To/1
  Sum/1 -> Math Function/1
  Min RPM/1 -> Sum/2
  MaxRPM/1 -> Sum/1
  Th K/1 -> Sum1/1
  dt/1 -> Saturation/1
  Sum1/1 -> MaxRPM/1
  Min Th K/1 -> Sum1/2

== system HILModel/Plant Model/Plant/Forces and Moments/Alpha/Beta ==
  "Vx, Vy, Vz (Body)" : Inport
  Rho : Inport  Port=2
  Constant : Constant  Value=0.5  VectorParams1D=off
  Math Function : Math  Operator=sqrt  SaturateOnIntegerOverflow=on
  Product : Product  Inputs=3  SaturateOnIntegerOverflow=on
  Product1 : Product  Inputs=3  SaturateOnIntegerOverflow=on
  R2D1 : Gain  Gain=180/pi  SaturateOnIntegerOverflow=on
  R2D2 : Gain  Gain=180/pi  SaturateOnIntegerOverflow=on
  V^2 : Fcn  Expr=(u(1)^2+u(2)^2+u(3)^2)
  "[-15; 15 ]" : Saturate  UpperLimit=15  LowerLimit=-15
  "[-15;15]" : Saturate  UpperLimit=15  LowerLimit=-15
  aoa : Trigonometry  Operator=asin
  beta : Trigonometry  Operator=atan
  sin(aoa) : Fcn  Expr=u(3)/sqrt(u(1)^2+u(3)^2)
  span : Constant  Value=span  VectorParams1D=off
  span1 : Constant  Value=chord  VectorParams1D=off
  tan(beta) : Fcn  Expr=u(2)/sqrt(u(1)^2+u(3)^2)
  "alpha, deg" : Outport
  "beta, deg" : Outport  Port=2
  qS : Outport  Port=3
  Speed : Outport  Port=4
  q : Outport  Port=5
  wires:
  Product/1 -> q/1, Product1/1
  Product1/1 -> qS/1
  span1/1 -> Product1/3
  span/1 -> Product1/2
  "Vx, Vy, Vz (Body)"/1 -> sin(aoa)/1, V^2/1, tan(beta)/1
  tan(beta)/1 -> beta/1
  beta/1 -> R2D1/1
  V^2/1 -> Product/1, Math Function/1
  Rho/1 -> Product/2
  Constant/1 -> Product/3
  R2D1/1 -> "[-15; 15 ]"/1  "beta"
  aoa/1 -> R2D2/1
  R2D2/1 -> "[-15;15]"/1  "aoa"
  sin(aoa)/1 -> aoa/1
  Math Function/1 -> Speed/1
  "[-15;15]"/1 -> "alpha, deg"/1
  "[-15; 15 ]"/1 -> "beta, deg"/1

== system HILModel/Plant Model/Plant/Forces and Moments/Body Frame F & M ==
  "Alpha, deg" : Inport
  "Beta, deg" : Inport  Port=2
  qs : Inport  Port=3
  Airspeed : Inport  Port=4
  "de, deg" : Inport  Port=5
  "da, deg" : Inport  Port=6
  "dr, deg" : Inport  Port=7
  "df, deg" : Inport  Port=8
  p,q,r : Inport  Port=9
  Bus Creator : BusCreator  Inputs=2
  Transfer to body frame : Subsystem
  Wind frame F& M : Subsystem
  F_b : Outport
  M_b : Outport  Port=2
  wires:
  "Alpha, deg"/1 -> Wind frame F& M/1("alpha, deg"), Bus Creator/1
  "Beta, deg"/1 -> Wind frame F& M/2("beta, deg"), Bus Creator/2
  "dr, deg"/1 -> Wind frame F& M/5("dr, deg")
  "da, deg"/1 -> Wind frame F& M/4("da, deg")
  "de, deg"/1 -> Wind frame F& M/3("de, deg")
  Wind frame F& M/1(F&M wind frame) -> Transfer to body frame/1(Wind frame  F&M)
  Bus Creator/1 -> Transfer to body frame/2("aoa/beta, deg")  "aoa/beta, deg"
  Transfer to body frame/1(F_b) -> F_b/1
  Transfer to body frame/2(M_b) -> M_b/1
  "df, deg"/1 -> Wind frame F& M/6("df, deg")
  qs/1 -> Wind frame F& M/7(qS)
  p,q,r/1 -> Wind frame F& M/8(p,q,r)
  Airspeed/1 -> Wind frame F& M/9(Airpseed)

== system HILModel/Plant Model/Plant/Forces and Moments/Get Grav Force in Body ==
  Euler : Inport
  Grav Force : Inport  Port=2
  Math Function : Math  Operator=transpose  SaturateOnIntegerOverflow=on
  Product1 : Product  Multiplication=Matrix(*)  SaturateOnIntegerOverflow=on  InputSameDT=on
  Rb2u : Subsystem
  Reshape : Reshape  OutputDimensionality=Column vector (2-D)
  Grav Force (Body) : Outport
  wires:
  Rb2u/1(DCM) -> Math Function/1
  Euler/1 -> Rb2u/1(phi theta psi)
  Product1/1 -> Grav Force (Body)/1
  Math Function/1 -> Product1/1
  Grav Force/1 -> Reshape/1
  Reshape/1 -> Product1/2

== system HILModel/Plant Model/Plant/Forces and Moments/NED(u)2b ==
  V w : Inport
  Euler : Inport  Port=2
  RB2LTP : Subsystem
  RL2B * Vw : Product  Multiplication=Matrix(*)  SaturateOnIntegerOverflow=on  InputSameDT=on
  RLTP2B : Math  Operator=transpose  SaturateOnIntegerOverflow=on
  Reshape1 : Reshape  OutputDimensionality=Row vector (2-D)
  Vb Corr : Outport
  wires:
  RL2B * Vw/1 -> Reshape1/1
  Euler/1 -> RB2LTP/1(Euler)
  RB2LTP/1(RB2L) -> RLTP2B/1
  RLTP2B/1 -> RL2B * Vw/1
  V w/1 -> RL2B * Vw/2
  Reshape1/1 -> Vb Corr/1

== system HILModel/Plant Model/Plant/Magnetometer/RB2LTP ==
  Euler : Inport
  11 : Fcn  Expr=cos(u[3])*cos(u[2])
  12 : Fcn  Expr=sin(u[3])*cos(u[2])
  13 : Fcn  Expr=-sin(u[2])
  21 : Fcn  Expr=cos(u[3])*sin(u[2])*sin(u[1])-sin(u[3])*cos(u[1])
  22 : Fcn  Expr=sin(u[3])*sin(u[2])*sin(u[1])+cos(u[3])*cos(u[1])
  23 : Fcn  Expr=cos(u[2])*sin(u[1])
  31 : Fcn  Expr=cos(u[3])*sin(u[2])*cos(u[1])+sin(u[3])*sin(u[1])
  32 : Fcn  Expr=sin(u[3])*sin(u[2])*cos(u[1])-cos(u[3])*sin(u[1])
  33 : Fcn  Expr=cos(u[2])*cos(u[1])
  Mux2 : Mux  Inputs=9
  Reshape : Reshape  OutputDimensionality=Customize  OutputDimensions=[3,3]
  Rot : Outport
  wires:
  33/1 -> Mux2/9
  32/1 -> Mux2/8
  31/1 -> Mux2/7
  23/1 -> Mux2/6
  22/1 -> Mux2/5
  21/1 -> Mux2/4
  13/1 -> Mux2/3
  12/1 -> Mux2/2
  11/1 -> Mux2/1
  Mux2/1 -> Reshape/1
  Euler/1 -> 11/1, 33/1, 32/1, 31/1, 23/1, 22/1, 21/1, 13/1, 12/1
  Reshape/1 -> Rot/1

== system HILModel/Plant Model/Plant/Wrap Around PSI1/Negative Yaw ==
  yaw : Inport
  Enable : EnablePort
  Abs : Abs
  Constant1 : Constant  Value=2*pi
  Constant2 : Constant  Value=2*pi
  Math Function : Math  Operator=mod  SaturateOnIntegerOverflow=on
  Sum : Sum  Inputs=|-+
  yaw_wr : Outport
  wires:
  yaw/1 -> Abs/1
  Constant1/1 -> Math Function/2
  Math Function/1 -> Sum/1
  Abs/1 -> Math Function/1
  Constant2/1 -> Sum/2
  Sum/1 -> yaw_wr/1

== system HILModel/Plant Model/Plant/Wrap Around PSI1/Positive Yaw ==
  yaw : Inport
  Enable : EnablePort
  Constant1 : Constant  Value=2*pi
  Math Function : Math  Operator=mod  SaturateOnIntegerOverflow=on
  yaw_wr : Outport
  wires:
  yaw/1 -> Math Function/1
  Constant1/1 -> Math Function/2
  Math Function/1 -> yaw_wr/1

== system HILModel/Plant Model/Subsystem/Three-Axis Magnetometer/Generic Sensor ==
  Sens : Inport
  Dynamics : Subsystem
  Measurement bias : Constant  Value=g_bias
  Product : Product  Multiplication=Matrix(*)  SaturateOnIntegerOverflow=on
  Random bias : simulink/Sources/Band-Limited White Noise  SystemSampleTime=-1  Cov=g_pow  Ts=g_Ts  seed=g_seeds(1:3)
  Saturation : Saturate  UpperLimit=g_sat(4:6)  LowerLimit=g_sat(1:3)
  "Scale factors & Cross-coupling  errors " : Constant  Value=g_sf_cc
  Sum1 : Sum  Inputs=|++  SaturateOnIntegerOverflow=on
  Sum4 : Sum  Inputs=++|  SaturateOnIntegerOverflow=on
  Zero-Order Hold : ZeroOrderHold  SampleTime=g_Ts
  Meas : Outport
  wires:
  Zero-Order Hold/1 -> Product/2
  Dynamics/1(Sens Dyn) -> Sum1/1
  Sum1/1 -> Saturation/1
  Sens/1 -> Zero-Order Hold/1
  Saturation/1 -> Meas/1
  Random bias/1 -> Sum1/2
  "Scale factors & Cross-coupling  errors "/1 -> Product/1
  Sum4/1 -> Dynamics/1("Sens ")
  Product/1 -> Sum4/1
  Measurement bias/1 -> Sum4/2

== system HILModel/Autopilot/Autopilot/Altitude Control Vector Inputs/PID Controller/Extended Integrator ==
  note: Trapezoidal integration with integrator reset and anti-windup logic
      | The block computes the integral.  The integrator gets the IC value
      | whenever the enable line is down.  Anytime the enable line is
      | down the output is the IC value.  If the gain goes to zero then the
      | integrator value is reset.
  note: Trapezoidal multiplication based upon taking
      | the average of the previous and current inputs
  note: Integral summation
  Input : Inport
  IniCond : Inport  Port=2
  Enable : Inport  Port=3
  Gain : Inport  Port=4
  Limits : Inport  Port=5
  Apply Gain : Product  SaturateOnIntegerOverflow=on  InputSameDT=on
  Enable detect : Switch  Threshold=0.5  SaturateOnIntegerOverflow=on  InputSameDT=on
  Is gain zero? : RelationalOperator  Operator===  InputSameDT=on
  Previous Input : Memory  InheritSampleTime=on
  Previous State : Memory  Orientation=left  InheritSampleTime=on
  SaturationEx : piccolo_library/Nonlinear/SaturationEx  SystemSampleTime=-1
  Sum1 : Sum  SaturateOnIntegerOverflow=on  InputSameDT=on
  Sum2 : Sum  SaturateOnIntegerOverflow=on  InputSameDT=on
  T/2 : Gain  Gain=0.5*T
  Zero : Constant  Value=0
  Zero gain detect : Switch  Threshold=0.5  SaturateOnIntegerOverflow=on  InputSameDT=on
  Out : Outport  OutDataType=fixdt(1,16,0)  OutScaling=[]
  wires:
  SaturationEx/1 -> Out/1, Previous State/1
  Limits/1 -> SaturationEx/2
  Zero gain detect/1 -> SaturationEx/1
  Enable detect/1 -> Zero gain detect/3
  Is gain zero?/1 -> Zero gain detect/2
  Enable/1 -> Enable detect/2
  IniCond/1 -> Zero gain detect/1, Enable detect/3
  Sum1/1 -> Enable detect/1
  Zero/1 -> Is gain zero?/2
  Previous State/1 -> Sum1/2
  Apply Gain/1 -> Sum1/1
  Gain/1 -> Is gain zero?/1, Apply Gain/2
  T/2/1 -> Apply Gain/1
  Sum2/1 -> T/2/1
  Input/1 -> Previous Input/1, Sum2/1
  Previous Input/1 -> Sum2/2

== system HILModel/Autopilot/Autopilot/Guidance & Navigation Vector Input/Wind-relative Tracker/K Schedule ==
  note: Schedule K to provide a tighter convergence as the cross track parameter Y gets small.
      | Use the formula K = K((1-b)*sin(PI*Y/2/K) + b); the scaling only applies when Y is less than K
  K in : Inport
  Y : Inport  Port=2
  Abs : Abs  SaturateOnIntegerOverflow=on
  If : If  NumInputs=2  IfExpression=u1<u2
  If Y is less than K : Subsystem  TreatAsAtomicUnit=on
  If Yis greater than K : Subsystem  TreatAsAtomicUnit=on
  Merge : Merge
  K out : Outport  OutDataType=fixdt(1,16,0)  OutScaling=[]
  wires:
  If/1 -> If Yis greater than K/Action
  If/2 -> If Y is less than K/Action
  Y/1 -> Abs/1
  K in/1 -> If Y is less than K/1(K in), If/1, If Yis greater than K/1(In)
  Merge/1 -> K out/1
  If Yis greater than K/1(Out) -> Merge/1
  If Y is less than K/1(K out) -> Merge/2
  Abs/1 -> If/2, If Y is less than K/2(Y)

== system HILModel/Autopilot/Autopilot/Pitch Control  Vector Inputs/Pdyn Hold/PID Controller ==
  note: Standard PID feedback controller with integrator saturation. There are three gains, and three states, one for each term
  Input : Inport
  Cmd : Inport  Port=2
  State : Inport  Port=3
  Gains : Inport  Port=4
  Limits : Inport  Port=5
  IniCond : Inport  Port=6
  Demux : Demux  Outputs=3
  Demux1 : Demux  Outputs=3
  Derivative Gain : Product  Inputs=3  SaturateOnIntegerOverflow=on  InputSameDT=on
  Extended Integrator : piccolo_library/Integrators/Extended Integrator  SystemSampleTime=-1  T=tsamp
  Proportional Gain : Product  Inputs=3  SaturateOnIntegerOverflow=on  InputSameDT=on
  Scope3 : Scope  NumInputPorts=3
      settings: YMin=-0.045~-1~-1  YMax=-0.0075~1~1  SaveName=ScopeData21
  Sum : Sum  Inputs=|+-  SaturateOnIntegerOverflow=on
  Sum3 : Sum  Inputs=+++  SaturateOnIntegerOverflow=on  InputSameDT=on
  dx/dt with TD : piccolo_library/Derivatives/dx//dt with TD  SystemSampleTime=-1  tsamp=tsamp  tdelay=tdelay
  Output : Outport  OutDataType=fixdt(1,16,0)  OutScaling=[]
  wires:
  Sum3/1 -> Output/1
  Demux1/3 -> Derivative Gain/3
  Demux1/2 -> Extended Integrator/3
  Demux1/1 -> Proportional Gain/3
  State/1 -> Demux1/1
  IniCond/1 -> Extended Integrator/2
  Limits/1 -> Extended Integrator/5
  Demux/2 -> Extended Integrator/4
  Extended Integrator/1 -> Sum3/2, Scope3/2
  Derivative Gain/1 -> Sum3/3, Scope3/3
  Proportional Gain/1 -> Sum3/1, Scope3/1
  Demux/3 -> Derivative Gain/2
  Demux/1 -> Proportional Gain/2
  Gains/1 -> Demux/1
  dx/dt with TD/1 -> Derivative Gain/1
  Sum/1 -> Extended Integrator/1, dx/dt with TD/1, Proportional Gain/1
  Cmd/1 -> Sum/2
  Input/1 -> Sum/1
